simulink model "movingAverage"  (R2022b)
settings: Solver=FixedStepDiscrete  StartTime=t(1)  StopTime=t(end)  RelTol=1e-3  EnableMultiTasking=on
PreLoadFcn:
  | % Load data from file
  | data = readmatrix("temp.xls");
  | t = data(:,1);
  | u = data(:,2);
settings Model: Creator=jrivitus  LastModifiedBy=bensweet
settings SolverCC: AlgebraicLoopSolver=TrustRegion
settings DataIOCC: LimitDataPoints=on  LoadExternalInput=on  SaveFormat=Array  ReturnWorkspaceOutputs=off
settings OptimizationCC: ExpressionDepthLimit=2147483647  InitFltsAndDblsToZero=on  LifeSpan=inf
settings DebuggingCC: UnconnectedInputMsg=warning  UnconnectedOutputMsg=warning  UnconnectedLineMsg=warning  PregeneratedLibrarySubsystemCodeDiagnostic=none  SFMachineParentedDataDiag=warning
settings HardwareCC: ProdBitPerPointer=32  ProdBitPerSizeT=32  ProdBitPerPtrDiffT=32  ProdLargestAtomicFloat=None  ProdIntDivRoundTo=Undefined  ProdEndianess=Unspecified  ProdWordSize=32  ProdHWDeviceType=32-bit Generic
settings ModelReferenceCC: EnableRefExpFcnMdlSchedulingChecks=on  PropagateSignalLabelsOutOfModel=off
settings SFSimCC: SimUseLocalCustomCode=off
settings RTWCC: RTWUseLocalCustomCode=off  DLArmComputeVersion=19.05
settings CodeAppCC: StateflowObjectComments=on
settings GRTTargetCC: TargetLangStandard=C89/C90 (ANSI)  CombineOutputUpdateFcns=off  GRTInterface=on
settings ConfigComp: CovMetricSettings=dw  CovSaveCumulativeToWorkspaceVar=on  CovSaveSingleToWorkspaceVar=on  CovExternalEMLEnable=off  CovSFcnEnable=off

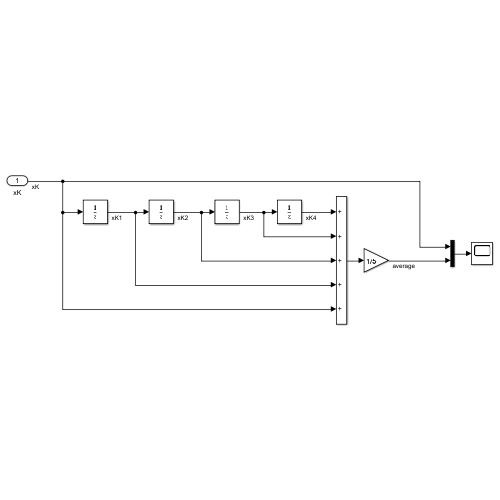
[thumbnail: Simulink's stored preview of the top-level diagram]
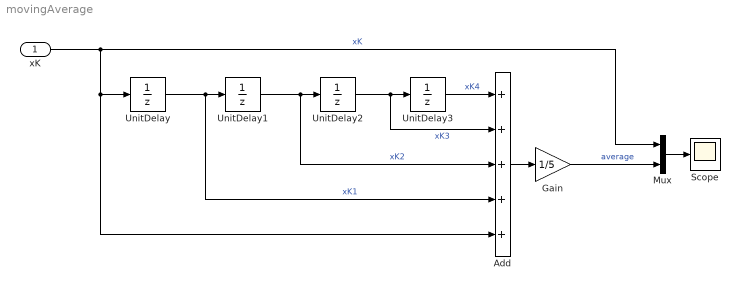
== system movingAverage ==
  xK : Inport
  Add : Sum  Inputs=+++++
  Gain : Gain  Gain=1/5
  Mux : Mux  Inputs=2
  Scope : Scope
  UnitDelay{,1..3} (4 alike) : UnitDelay  HasFrameUpgradeWarning=on
  wires:
  xK/1 -> Mux/1, Add/5, UnitDelay/1  "xK"
  UnitDelay/1 -> UnitDelay1/1, Add/4  "xK1"
  UnitDelay1/1 -> UnitDelay2/1, Add/3  "xK2"
  UnitDelay2/1 -> UnitDelay3/1, Add/2  "xK3"
  UnitDelay3/1 -> Add/1  "xK4"
  Add/1 -> Gain/1
  Gain/1 -> Mux/2  "average"
  Mux/1 -> Scope/1
